simulink model "simulator_in_the_loop"  (R2025a)
settings: Solver=VariableStepAuto  StartTime=0.0  StopTime=0.5  FixedStep=1e-6  RelTol=1e-3
libraries: instrumentlib x3, mcbplantlib x1, mcbpositiondecoderlib x1, mcbcontrolslib x1, autolibpmsmexterior x1
settings Model: Creator=brandon  LastModifiedBy=brandon

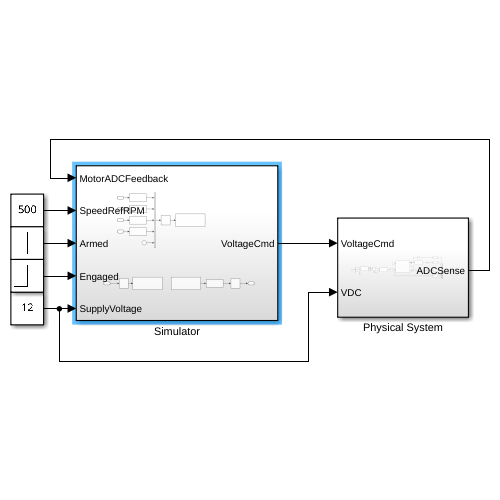
[thumbnail: Simulink's stored preview of the top-level diagram]
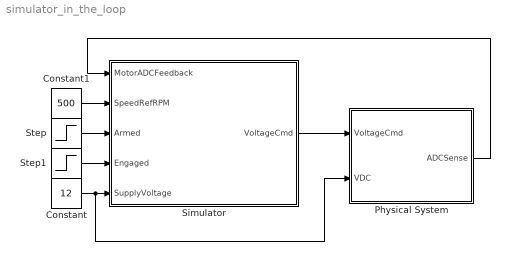
== system simulator_in_the_loop ==
  Constant : Constant  Value=12
  Constant1 : Constant  Value=500
  Physical System : Subsystem
  Simulator : Subsystem
  Step : Step  Time=0.05  SampleTime=0
  Step1 : Step  Time=0.15  SampleTime=0
  wires:
  Simulator/1(VoltageCmd) -> Physical System/1(VoltageCmd)
  Physical System/1(ADCSense) -> Simulator/1(MotorADCFeedback)
  Constant1/1 -> Simulator/2(SpeedRefRPM)
  Constant/1 -> Physical System/2(VDC), Simulator/5(SupplyVoltage)
  Step1/1 -> Simulator/4(Engaged)
  Step/1 -> Simulator/3(Armed)

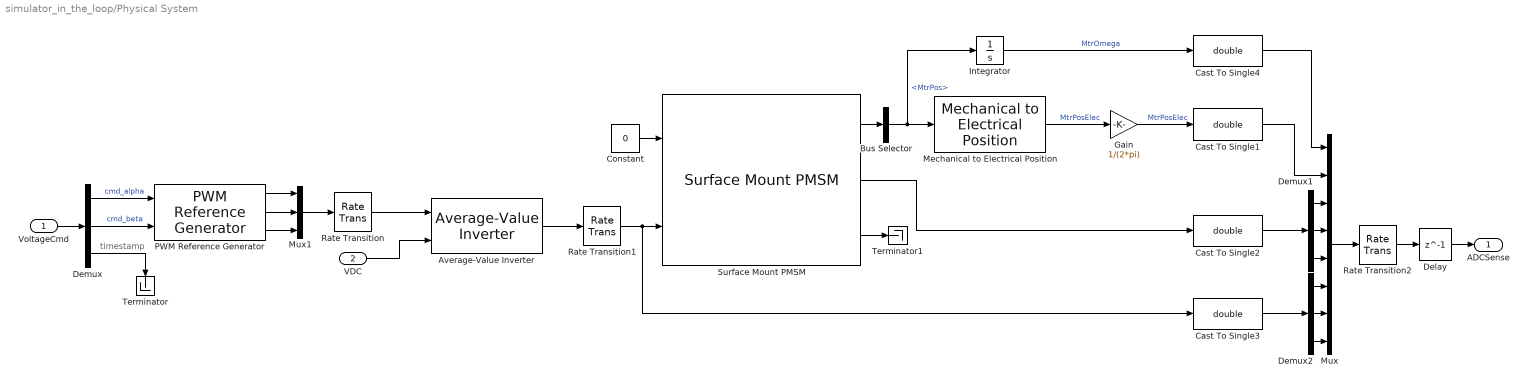
== system simulator_in_the_loop/Physical System ==
  note: timestamp
  VoltageCmd : Inport
  VDC : Inport  Port=2
  Average-Value Inverter : mcbplantlib/Average-Value Inverter
      settings: LibrarySourceBlock=mcblib/Electrical Systems/Inverters/Average-Value Inverter
  Bus Selector : BusSelector  OutputSignals=MtrPos
  Cast To Single{1..4} (4 alike) : DataTypeConversion  OutDataTypeStr=double  SaturateOnIntegerOverflow=off  RndMeth=Floor
  Constant : Constant  Value=0
  Delay : Delay  DelayLength=1
  Demux : Demux  Outputs=3
  Demux1 : Demux  Outputs=3
  Demux2 : Demux  Outputs=3
  Gain : Gain  Gain=1/(2*pi)  OutDataTypeStr=Inherit: Same as input
  Integrator : Integrator
  Mechanical to Electrical Position : mcbpositiondecoderlib/Mechanical to Electrical Position  PolePairsInputType=Specify via dialog  NrPP=7  selectedRange=Radians  MechOfstInputType=Specify via dialog  mechOffsetIn=0  maxAngleIn=2*pi  InputDataType=single  VariantSelect=floating-point
  Mux : Mux  Inputs=8
  Mux1 : Mux  Inputs=3
  PWM Reference Generator : mcbcontrolslib/PWM Reference Generator  inSignal=Valphabeta  modType=SVM: space vector modulation
      settings: LibrarySourceBlock=mcblib/Controls/Math Transforms/PWM Reference Generator
  Rate Transition : RateTransition
  Rate Transition1 : RateTransition
  Rate Transition2 : RateTransition
  Surface Mount PMSM : autolibpmsmexterior/Surface Mount PMSM  port_config=Torque  sim_type=Discrete  Ts=0.001  P=7  Rs=0.02  Ldq_=1.7e-3  KConstText=Permanent flux linkage constant (lambda_pm):  lambda_pm=0.2205  Ke=159.9771  Kt=1.323  mechanical=[0.0027, 4.924e-4, 0]  idq0=[0 0]  theta_init=0  omega_init=0  KConst=0.2205  lambda_pm_calc=0.2205  RefBlkName='autolibpmsmexterior/Surface Mount PMSM'  aMode=5  Ldq="[0.0017      0.0017]"
  Terminator : Terminator
  Terminator1 : Terminator
  ADCSense : Outport
  wires:
  VoltageCmd/1 -> Demux/1
  Demux/2 -> PWM Reference Generator/2  "cmd_beta"
  Demux/1 -> PWM Reference Generator/1  "cmd_alpha"
  Demux/3 -> Terminator/1
  PWM Reference Generator/1 -> Mux1/1
  PWM Reference Generator/2 -> Mux1/2
  PWM Reference Generator/3 -> Mux1/3
  VDC/1 -> Average-Value Inverter/2
  Mux1/1 -> Rate Transition/1
  Rate Transition/1 -> Average-Value Inverter/1
  Average-Value Inverter/1 -> Rate Transition1/1
  Surface Mount PMSM/3 -> Terminator1/1
  Surface Mount PMSM/1 -> Bus Selector/1
  Bus Selector/1 -> Integrator/1, Mechanical to Electrical Position/1  "<MtrPos>"
  Mechanical to Electrical Position/1 -> Gain/1  "MtrPosElec"
  Gain/1 -> Cast To Single1/1  "MtrPosElec"
  Cast To Single2/1 -> Demux1/1
  Cast To Single3/1 -> Demux2/1
  Rate Transition1/1 -> Surface Mount PMSM/2, Cast To Single3/1
  Surface Mount PMSM/2 -> Cast To Single2/1
  Constant/1 -> Surface Mount PMSM/1
  Mux/1 -> Rate Transition2/1
  Rate Transition2/1 -> Delay/1
  Delay/1 -> ADCSense/1
  Demux1/1 -> Mux/3
  Demux1/2 -> Mux/4
  Demux1/3 -> Mux/5
  Demux2/1 -> Mux/6
  Demux2/2 -> Mux/7
  Demux2/3 -> Mux/8
  Cast To Single1/1 -> Mux/2
  Cast To Single4/1 -> Mux/1
  Integrator/1 -> Cast To Single4/1  "MtrOmega"

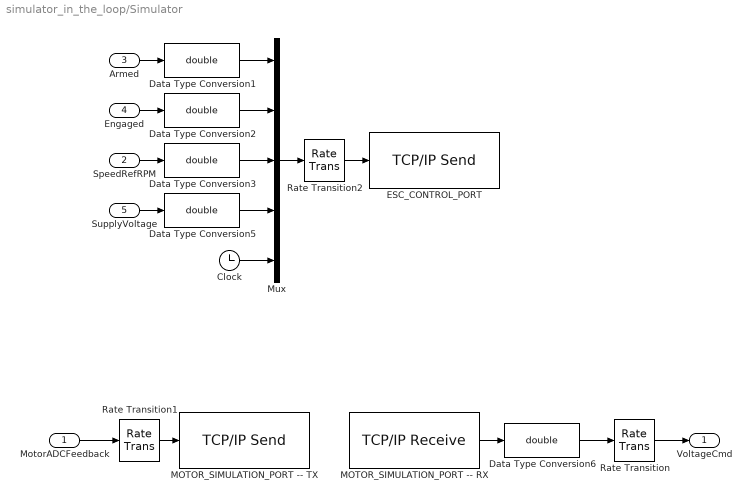
== system simulator_in_the_loop/Simulator ==
  MotorADCFeedback : Inport
  SpeedRefRPM : Inport  Port=2
  Armed : Inport  Port=3
  Engaged : Inport  Port=4
  SupplyVoltage : Inport  Port=5
  Clock : Clock
      settings: Decimation=12
  Data Type Conversion{1..3,5..6} (5 alike) : DataTypeConversion  OutDataTypeStr=double  SaturateOnIntegerOverflow=off  RndMeth=Floor
  ESC_CONTROL_PORT : instrumentlib/TCP//IP Send  Priority=1  Host=localhost  Port=55003  ByteOrder=little-endian  EnableBlockingMode=on  Timeout=180  TransferDelay=on  SimulateUsing=Interpreted execution
  "MOTOR_SIMULATION_PORT -- RX" : instrumentlib/TCP//IP Receive  Priority=3  Host=localhost  Port=55001  DataSize=[ 3, 1 ]  DataType=single  ASCIIFormatting=%f  Terminator=LF  CustomTerminator=10  ByteOrder=little-endian  EnableBlockingMode=on  Timeout=180  SampleTime=0.00005  SimulateUsing=Interpreted execution
  "MOTOR_SIMULATION_PORT -- TX" : instrumentlib/TCP//IP Send  Priority=2  Host=localhost  Port=55001  ByteOrder=little-endian  EnableBlockingMode=on  Timeout=180  TransferDelay=on  SimulateUsing=Interpreted execution
  Mux : Mux  Inputs=5
  Rate Transition : RateTransition
  Rate Transition1 : RateTransition
  Rate Transition2 : RateTransition
  VoltageCmd : Outport
  wires:
  Data Type Conversion3/1 -> Mux/3
  Data Type Conversion5/1 -> Mux/4
  Data Type Conversion2/1 -> Mux/2
  Data Type Conversion1/1 -> Mux/1
  SupplyVoltage/1 -> Data Type Conversion5/1
  SpeedRefRPM/1 -> Data Type Conversion3/1
  Armed/1 -> Data Type Conversion1/1
  Engaged/1 -> Data Type Conversion2/1
  Clock/1 -> Mux/5
  "MOTOR_SIMULATION_PORT -- RX"/1 -> Data Type Conversion6/1
  Data Type Conversion6/1 -> Rate Transition/1
  Rate Transition/1 -> VoltageCmd/1
  Rate Transition1/1 -> "MOTOR_SIMULATION_PORT -- TX"/1
  MotorADCFeedback/1 -> Rate Transition1/1
  Mux/1 -> Rate Transition2/1
  Rate Transition2/1 -> ESC_CONTROL_PORT/1
